simulink model "Neurofeedback_Fuzzy_MISO_Full_3x3"  (R2022a)
settings: Solver=VariableStepAuto  StartTime=0.0  StopTime=2700  RelTol=1e-3
libraries: dspsrcs4 x12, simulink x5, fuzblock x1
(part 1 of 2)
settings Model: Creator=mdls3  LastModifiedBy=mariodelossantos
settings DebuggingCC: SignalRangeChecking=warning  UnderSpecifiedDimensionMsg=warning

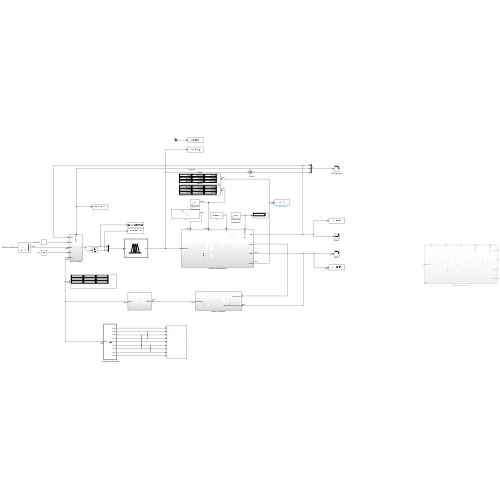
[thumbnail: Simulink's stored preview of the top-level diagram]
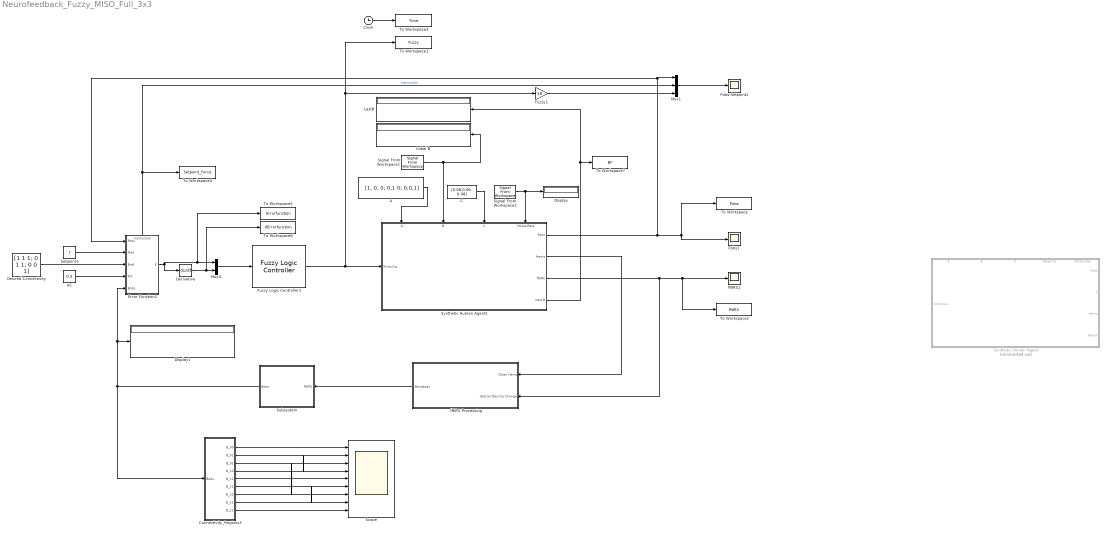
== system Neurofeedback_Fuzzy_MISO_Full_3x3 ==
  A : Constant  Value=[1, 0, 0; 0,1 0; 0,0,1]
  C : Constant  Value=[0.08;0.06; 0.08]
  Clock : Clock
  Connectivity_Regions3 : MATLAB Function  TreatAsAtomicUnit=on
  Derivative : Derivative  CoefficientInTFapproximation=1
  Desired Connectivity : Constant  Value="[1   1  1; 0 1 1; 0 0 1]"
  Display : Display
  Display1 : Display
  Error Function2 : Subsystem
      settings: PortSchema="{\"entries\":[{\"content\":{\"sides\":[{\"content\":{\"connectorIds\":[\"In1\",\"In2\",\"In3\",\"In4\",\"In5\"]},\"type\":\"ConnectorPlacement.EquallySpacedRectSide\",\"uuid\":\"444fbf9f-83f0-405e-b780-73f2a519e5d8\"},{\"content\":{\"connectorIds\":[\"Out1\"],\"side\":\"RIGHT\"},\"type\":\"ConnectorPlacement.EquallySpacedRectSide\",\"uuid\":\"580feeb9-eb76-4e38-ada2-7c0fba9b3602\"},{\"content\":{\"connectorIds\":[\"Out2\"],\"side\":\"TOP\"},\"type\":\"ConnectorPlacement.EquallySpacedRectSide\",\"uuid\":\"86f5bef5-f023-4b75-b93f-dc016b73225e\"}]},\"type\":\"ConnectorPlacement.EquallySpacedConnector\",\"uuid\":\"50bb9fda-b7f3-427b-ab4c-df885dc392aa\"}],\"packageUris\":[\"http://schema.mathworks.com/mf0/Connector/R2020b\"],\"version\":\"1.0\"}"
  Fuzzy Logic Controller1 : fuzblock/Fuzzy Logic  Controller  FIS=cFNIRS_MISO_v4  OutputSampleNumber=101  DataType=double  FuzzifiedInputs=off  RuleFiringStrengths=off  RuleOutputs=off  AggregatedOutputs=off  SimulateUsing=Interpreted execution  OutOfRangeInputValueMessage=warning  NoRuleFiredMessage=warning  EmptyOutputFuzzySetMessage=warning
  Fuzzy1 : Gain  Gain=10
  Initial B : Display
  LastB : Display
  Mux1 : Mux  Inputs=3
  Mux4 : Mux  Inputs=2
  Pobs-Setpoint1 : Scope
  Pobs1 : Scope
  Scope : Scope  NumInputPorts=9
  Setpoint1 : Constant  Value=7
  Signal From Workspace1 : dspsrcs4/Signal From Workspace  X=B  Ts=1  nsamps=1  OutputAfterFinalValue=Setting to zero  ignoreOrWarnInputAndFrameLengths=off  OutputFrames=off
  Signal From Workspace2 : dspsrcs4/Signal From Workspace  X=Noise  Ts=1  nsamps=1  OutputAfterFinalValue=Setting to zero  ignoreOrWarnInputAndFrameLengths=off  OutputFrames=off
  Subsystem : Subsystem
  Synthetic Human Agent : Subsystem  Commented=on
      settings: PortSchema="{\"entries\":[{\"content\":{\"sides\":[{\"content\":{\"connectorIds\":[\"In1\"]},\"type\":\"ConnectorPlacement.EquallySpacedRectSide\",\"uuid\":\"bfbcc5e8-6241-430f-b542-d1842988c81e\"},{\"content\":{\"connectorIds\":[\"Out1\",\"Out2\",\"Out3\",\"Out4\"],\"side\":\"RIGHT\"},\"type\":\"ConnectorPlacement.EquallySpacedRectSide\",\"uuid\":\"5787ae13-1686-4c0f-bd71-92bd424cb6c3\"},{\"content\":{\"connectorIds\":[\"In2\",\"In3\",\"In4\",\"In5\",\"In6\"],\"side\":\"TOP\"},\"type\":\"ConnectorPlacement.EquallySpacedRectSide\",\"uuid\":\"d1dd531e-b262-408a-a912-471f5b03e825\"}]},\"type\":\"ConnectorPlacement.EquallySpacedConnector\",\"uuid\":\"b2c21004-90c2-4258-a219-9564d29dafe7\"}],\"packageUris\":[\"http://schema.mathworks.com/mf0/Connector/R2020b\"],\"version\":\"1.0\"}"
  Synthetic Human Agent1 : Subsystem
      settings: PortSchema="{\"entries\":[{\"content\":{\"sides\":[{\"content\":{\"connectorIds\":[\"In1\"]},\"type\":\"ConnectorPlacement.EquallySpacedRectSide\",\"uuid\":\"bfbcc5e8-6241-430f-b542-d1842988c81e\"},{\"content\":{\"connectorIds\":[\"Out1\",\"Out2\",\"Out3\",\"Out4\"],\"side\":\"RIGHT\"},\"type\":\"ConnectorPlacement.EquallySpacedRectSide\",\"uuid\":\"5787ae13-1686-4c0f-bd71-92bd424cb6c3\"},{\"content\":{\"connectorIds\":[\"In2\",\"In3\",\"In4\",\"In5\"],\"side\":\"TOP\"},\"type\":\"ConnectorPlacement.EquallySpacedRectSide\",\"uuid\":\"d1dd531e-b262-408a-a912-471f5b03e825\"}]},\"type\":\"ConnectorPlacement.EquallySpacedConnector\",\"uuid\":\"b2c21004-90c2-4258-a219-9564d29dafe7\"}],\"packageUris\":[\"http://schema.mathworks.com/mf0/Connector/R2020b\"],\"version\":\"1.0\"}"
  To Workspace : ToWorkspace  VariableName=Pobs  SampleTime=-1
  To Workspace1 : ToWorkspace  VariableName=Fuzzy  SampleTime=-1
  To Workspace2 : ToWorkspace  VariableName=fNIRS  SampleTime=-1
  To Workspace3 : ToWorkspace  VariableName=Time  SampleTime=-1
      settings: Save2DSignal=2-D array (concatenate along first dimension)
  To Workspace4 : ToWorkspace  VariableName=Setpoint_Force  SampleTime=-1
  To Workspace5 : ToWorkspace  VariableName=Errorfunction  SampleTime=-1
  To Workspace6 : ToWorkspace  VariableName=dErrorfunction  SampleTime=-1
  To Workspace7 : ToWorkspace  VariableName=BF  SampleTime=-1
  fNIRS Processing : Subsystem
  fNIRS1 : Scope
  w1 : Constant  Value=0.5
  wires:
  Mux1/1 -> Pobs-Setpoint1/1
  Error Function2/1(E) -> Mux4/1, To Workspace5/1, Derivative/1
  Fuzzy1/1 -> Mux1/3
  Synthetic Human Agent1/2(Hemo) -> fNIRS Processing/1(Clean Hemo)
  Derivative/1 -> To Workspace6/1, Mux4/2
  Setpoint1/1 -> Error Function2/2(Pref)
  Error Function2/2(Instruction) -> Mux1/2, To Workspace4/1  "Instruction"
  Synthetic Human Agent1/1(Pobs) -> Error Function2/1(Pobs), Mux1/1, To Workspace/1, Pobs1/1
  Mux4/1 -> Fuzzy Logic Controller1/1
  A/1 -> Synthetic Human Agent1/2(A)
  w1/1 -> Error Function2/4(W1)
  Desired Connectivity/1 -> Error Function2/3(Bref)
  C/1 -> Synthetic Human Agent1/4(C)
  Fuzzy Logic Controller1/1 -> To Workspace1/1, Fuzzy1/1, Synthetic Human Agent1/1(Stimulus)
  Clock/1 -> To Workspace3/1
  Synthetic Human Agent1/4(New B) -> To Workspace7/1, LastB/1
  Signal From Workspace1/1 -> Initial B/1, Synthetic Human Agent1/3(B)
  Signal From Workspace2/1 -> Display/1, Synthetic Human Agent1/5(Noise-Rate)
  Subsystem/1(Bobs) -> Connectivity_Regions3/1(Bobs), Error Function2/5(Bobs), Display1/1
  Synthetic Human Agent1/3(fNIRS) -> fNIRS1/1, To Workspace2/1, fNIRS Processing/2(Optical Density Changes)
  Connectivity_Regions3/1(B_00) -> Scope/1
  Connectivity_Regions3/2(B_01) -> Scope/4
  Connectivity_Regions3/3(B_02) -> Scope/7
  Connectivity_Regions3/4(B_10) -> Scope/2
  Connectivity_Regions3/5(B_11) -> Scope/5
  Connectivity_Regions3/6(B_12) -> Scope/8
  Connectivity_Regions3/7(B_20) -> Scope/3
  Connectivity_Regions3/8(B_21) -> Scope/6
  Connectivity_Regions3/9(B_22) -> Scope/9
  fNIRS Processing/1(Bandpass) -> Subsystem/1(fNIRS)

== system Neurofeedback_Fuzzy_MISO_Full_3x3/Error Function2 ==
  Pobs : Inport
  Pref : Inport  Port=2
  Bref : Inport  Port=3
  W1 : Inport  Port=4
  Bobs : Inport  Port=5
  Error Function : Subsystem
  Rehabilitation Train : Subsystem
  E : Outport
  Instruction : Outport  Port=2
  wires:
  Bref/1 -> Error Function/3(Bref)
  Bobs/1 -> Error Function/4(Bobs)
  W1/1 -> Error Function/5(W1)
  Pref/1 -> Rehabilitation Train/1(In1)
  Pobs/1 -> Error Function/1(Pobs)
  Rehabilitation Train/1(Instruction) -> Instruction/1, Error Function/2(Pref)
  Error Function/1(E) -> E/1

== system Neurofeedback_Fuzzy_MISO_Full_3x3/Subsystem ==
  fNIRS : Inport
  DQ1 : Scope
  Incremental_Avg_Boot1 : Subsystem
  Threshold : Constant  Value=0.5
  getConnectivity_Validation1 : MATLAB Function  TreatAsAtomicUnit=on  SystemSampleTime=0
  Bobs : Outport
  wires:
  getConnectivity_Validation1/2(DQ) -> DQ1/1
  Incremental_Avg_Boot1/1("D ") -> getConnectivity_Validation1/1("D ")
  Threshold/1 -> getConnectivity_Validation1/2(Threshold)
  fNIRS/1 -> Incremental_Avg_Boot1/1(fNIRS)
  getConnectivity_Validation1/1(Bobs) -> Bobs/1

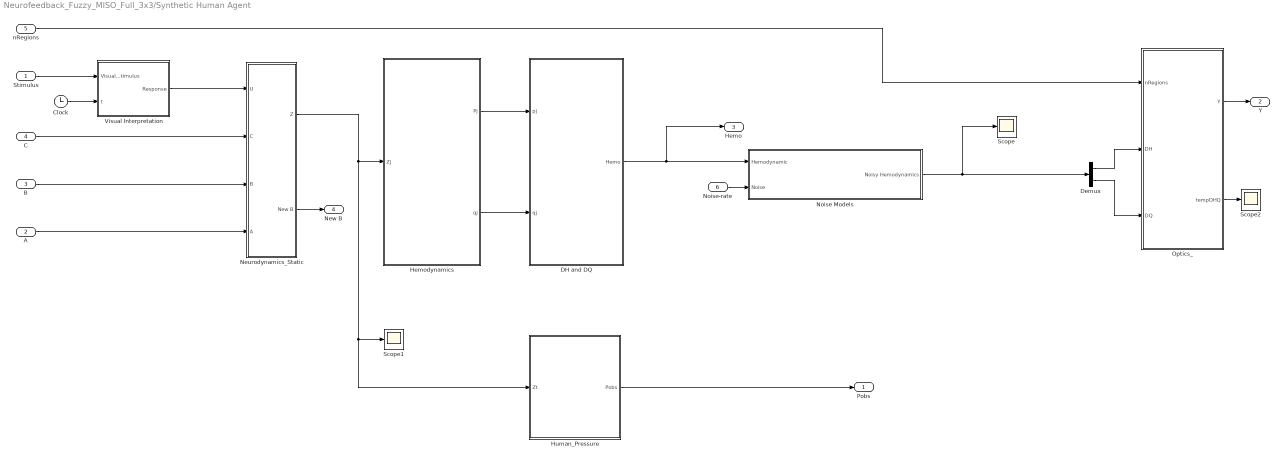
== system Neurofeedback_Fuzzy_MISO_Full_3x3/Synthetic Human Agent ==
  Stimulus : Inport
  A : Inport  Port=2
  B : Inport  Port=3
  C : Inport  Port=4
  nRegions : Inport  Port=5
  Noise-rate : Inport  Port=6
  Clock : Clock
  DH and DQ : Subsystem
  Demux : Demux  Outputs=2
  Hemodynamics : Subsystem
  Human_Pressure : Subsystem
  Neurodynamics_Static : Subsystem
  Noise Models : Subsystem
  Optics_ : MATLAB Function  TreatAsAtomicUnit=on
  Scope : Scope
  Scope1 : Scope
  Scope2 : Scope
  Visual Interpretation : MATLAB Function  TreatAsAtomicUnit=on
  Pobs : Outport
  Y : Outport  Port=2
  Hemo : Outport  Port=3
  New B : Outport  Port=4
  wires:
  DH and DQ/1(Hemo) -> Hemo/1, Noise Models/1(Hemodynamic)
  Hemodynamics/1(Pj) -> DH and DQ/1(pj)
  C/1 -> Neurodynamics_Static/2(C)
  Hemodynamics/2(qj) -> DH and DQ/2(qj)
  A/1 -> Neurodynamics_Static/4(A)
  Human_Pressure/1(Pobs) -> Pobs/1
  B/1 -> Neurodynamics_Static/3(B)
  Neurodynamics_Static/1(Z) -> Scope1/1, Human_Pressure/1(Zt), Hemodynamics/1(Zj)
  Clock/1 -> Visual Interpretation/2(t)
  Stimulus/1 -> Visual Interpretation/1(Visual_Stimulus)
  Visual Interpretation/1(Response) -> Neurodynamics_Static/1(U)
  Noise Models/1(Noisy Hemodynamics) -> Scope/1, Demux/1
  Noise-rate/1 -> Noise Models/2(Noise)
  Demux/1 -> Optics_/2(DH)
  Demux/2 -> Optics_/3(DQ)
  Optics_/1(Y) -> Y/1
  nRegions/1 -> Optics_/1(nRegions)
  Optics_/2(tempDHQ) -> Scope2/1
  Neurodynamics_Static/2(New B) -> New B/1

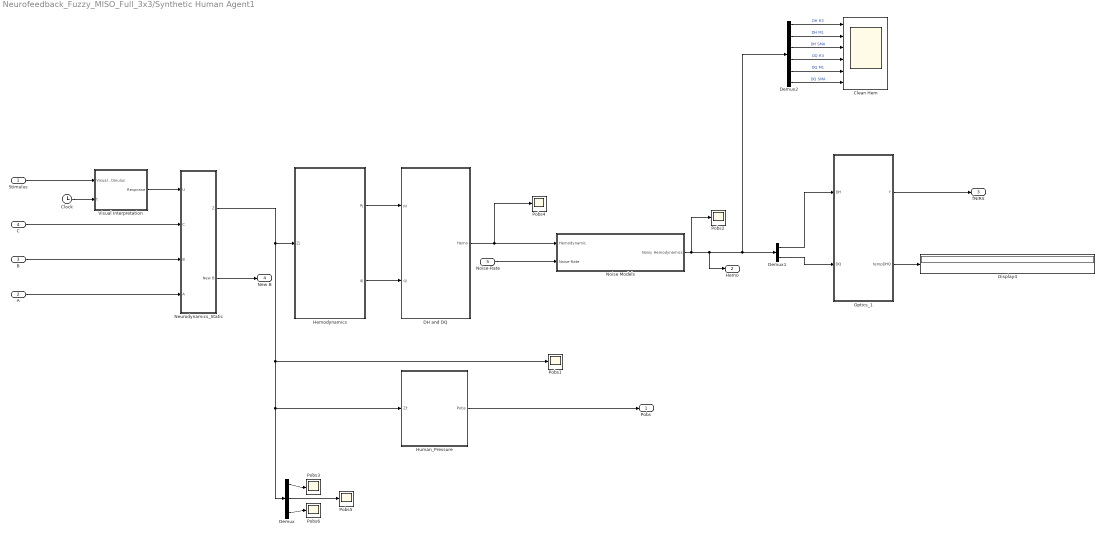
== system Neurofeedback_Fuzzy_MISO_Full_3x3/Synthetic Human Agent1 ==
  Stimulus : Inport
  A : Inport  Port=2
  B : Inport  Port=3
  C : Inport  Port=4
  Noise-Rate : Inport  Port=5
  Clean Hem : Scope  NumInputPorts=6
  Clock : Clock
  DH and DQ : Subsystem
  Demux : Demux  Outputs=3
  Demux1 : Demux  Outputs=2
  Demux2 : Demux  Outputs=6
  Display4 : Display
  Hemodynamics : Subsystem
  Human_Pressure : Subsystem
  Neurodynamics_Static : Subsystem
  Noise Models : Subsystem
  Optics_1 : MATLAB Function  TreatAsAtomicUnit=on
  Pobs{1..6} (6 alike) : Scope
  Visual Interpretation : MATLAB Function  TreatAsAtomicUnit=on
  Pobs : Outport
  Hemo : Outport  Port=2
  fNIRS : Outport  Port=3
  New B : Outport  Port=4
  wires:
  DH and DQ/1(Hemo) -> Pobs4/1, Noise Models/1(Hemodynamic)
  C/1 -> Neurodynamics_Static/2(C)
  A/1 -> Neurodynamics_Static/4(A)
  Human_Pressure/1(Pobs) -> Pobs/1
  B/1 -> Neurodynamics_Static/3(B)
  Demux1/1 -> Optics_1/1(DH)
  Demux1/2 -> Optics_1/2(DQ)
  Optics_1/1(Y) -> fNIRS/1
  Noise-Rate/1 -> Noise Models/2(Noise-Rate)
  Noise Models/1(Noisy Hemodynamics) -> Pobs2/1, Hemo/1, Demux2/1, Demux1/1
  Optics_1/2(tempDHQ) -> Display4/1
  Hemodynamics/1(Pj) -> DH and DQ/1(pj)
  Hemodynamics/2(qj) -> DH and DQ/2(qj)
  Demux2/2 -> Clean Hem/2  "DH M1"
  Demux2/1 -> Clean Hem/1  "DH R3"
  Demux2/3 -> Clean Hem/3  "DH SMA"
  Demux2/4 -> Clean Hem/4  "DQ R3"
  Demux2/5 -> Clean Hem/5  "DQ M1"
  Demux2/6 -> Clean Hem/6  "DQ SMA"
  Clock/1 -> Visual Interpretation/2(t)
  Stimulus/1 -> Visual Interpretation/1(Visual_Stimulus)
  Visual Interpretation/1(Response) -> Neurodynamics_Static/1(U)
  Neurodynamics_Static/2(New B) -> New B/1
  Demux/1 -> Pobs3/1
  Demux/2 -> Pobs5/1
  Demux/3 -> Pobs6/1
  Neurodynamics_Static/1(Z) -> Pobs1/1, Demux/1, Human_Pressure/1(Zt), Hemodynamics/1(Zj)

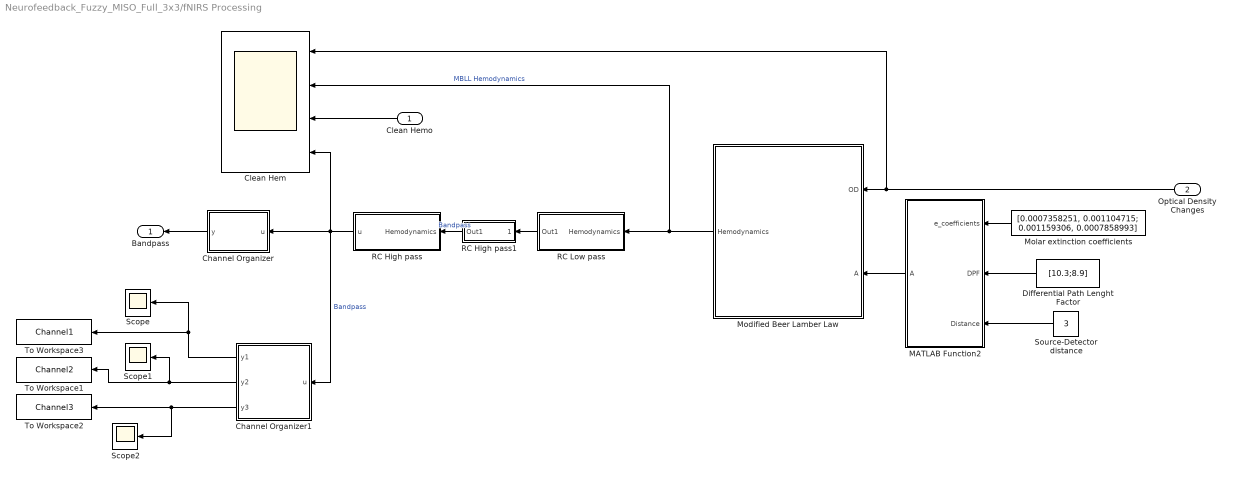
== system Neurofeedback_Fuzzy_MISO_Full_3x3/fNIRS Processing ==
  Clean Hemo : Inport
  Optical Density Changes : Inport  Port=2
  Channel Organizer : MATLAB Function  TreatAsAtomicUnit=on
  Channel Organizer1 : MATLAB Function  TreatAsAtomicUnit=on
  Clean Hem : Scope  NumInputPorts=4
  Differential Path Lenght Factor : Constant  Value=[10.3;8.9]
  MATLAB Function2 : MATLAB Function  TreatAsAtomicUnit=on
  Modified Beer Lamber Law : MATLAB Function  TreatAsAtomicUnit=on
  Molar extinction coefficients : Constant  Value=|
      | [0.0007358251, 0.001104715;
      | 0.001159306, 0.0007858993]
  RC High pass : Subsystem
  RC High pass1 : Subsystem
  RC Low pass : Subsystem
  Scope : Scope
  Scope1 : Scope
  Scope2 : Scope
  Source-Detector distance : Constant  Value=3
  To Workspace1 : ToWorkspace  VariableName=Channel2  SaveFormat=Structure With Time  SampleTime=-1
  To Workspace2 : ToWorkspace  VariableName=Channel3  SaveFormat=Structure With Time  SampleTime=-1
  To Workspace3 : ToWorkspace  VariableName=Channel1  SaveFormat=Structure With Time  SampleTime=-1
  Bandpass : Outport
  wires:
  Modified Beer Lamber Law/1(Hemodynamics) -> RC Low pass/1(Hemodynamics), Clean Hem/2  "MBLL Hemodynamics"
  Optical Density Changes/1 -> Clean Hem/1, Modified Beer Lamber Law/1(OD)
  RC High pass/1(u) -> Channel Organizer/1(u), Channel Organizer1/1(u), Clean Hem/4  "Bandpass"
  MATLAB Function2/1(A) -> Modified Beer Lamber Law/2(A)
  RC Low pass/1(Out1) -> RC High pass1/1(Hemodynamics)
  Clean Hemo/1 -> Clean Hem/3
  RC High pass1/1(Out1) -> RC High pass/1(Hemodynamics)  "Bandpass"
  Channel Organizer1/1(y1) -> Scope/1, To Workspace3/1
  Channel Organizer1/2(y2) -> Scope1/1, To Workspace1/1
  Channel Organizer1/3(y3) -> Scope2/1, To Workspace2/1
  Source-Detector distance/1 -> MATLAB Function2/3(Distance)
  Differential Path Lenght Factor/1 -> MATLAB Function2/2(DPF)
  Molar extinction coefficients/1 -> MATLAB Function2/1(e_coefficients)
  Channel Organizer/1(y) -> Bandpass/1

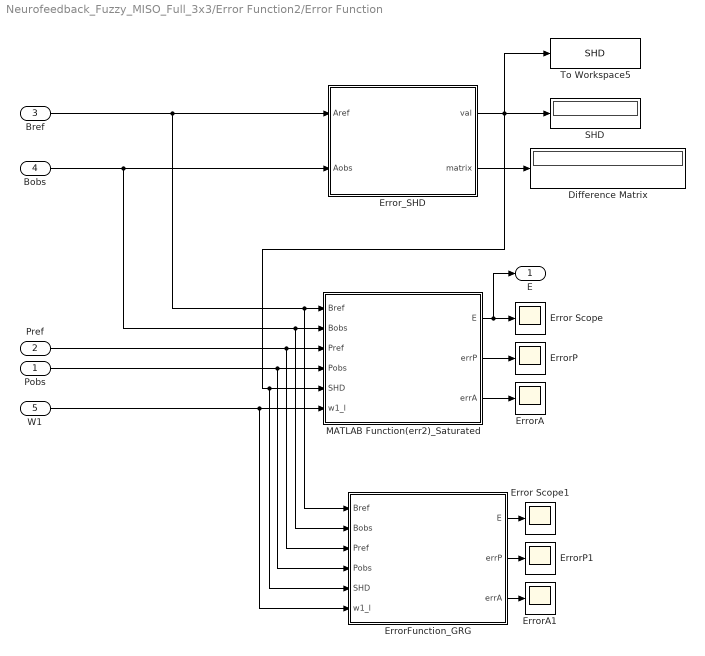
== system Neurofeedback_Fuzzy_MISO_Full_3x3/Error Function2/Error Function ==
  Pobs : Inport
  Pref : Inport  Port=2
  Bref : Inport  Port=3
  Bobs : Inport  Port=4
  W1 : Inport  Port=5
  Difference Matrix : Display
  Error Scope : Scope
  Error Scope1 : Scope
  ErrorA : Scope
  ErrorA1 : Scope
  ErrorFunction_GRG : MATLAB Function  TreatAsAtomicUnit=on
  ErrorP : Scope
  ErrorP1 : Scope
  Error_SHD : MATLAB Function  TreatAsAtomicUnit=on
  MATLAB Function(err2)_Saturated : MATLAB Function  TreatAsAtomicUnit=on
  SHD : Display
  To Workspace5 : ToWorkspace  VariableName=SHD  SampleTime=-1
  E : Outport
  wires:
  Error_SHD/2(matrix) -> Difference Matrix/1
  Bref/1 -> ErrorFunction_GRG/1(Bref), MATLAB Function(err2)_Saturated/1(Bref), Error_SHD/1(Aref)
  Error_SHD/1(val) -> To Workspace5/1, ErrorFunction_GRG/5(SHD), MATLAB Function(err2)_Saturated/5(SHD), SHD/1
  Bobs/1 -> ErrorFunction_GRG/2(Bobs), MATLAB Function(err2)_Saturated/2(Bobs), Error_SHD/2(Aobs)
  Pref/1 -> ErrorFunction_GRG/3(Pref), MATLAB Function(err2)_Saturated/3(Pref)
  W1/1 -> MATLAB Function(err2)_Saturated/6(w1_l), ErrorFunction_GRG/6(w1_l)
  MATLAB Function(err2)_Saturated/1(E) -> E/1, Error Scope/1
  Pobs/1 -> ErrorFunction_GRG/4(Pobs), MATLAB Function(err2)_Saturated/4(Pobs)
  MATLAB Function(err2)_Saturated/2(errP) -> ErrorP/1
  MATLAB Function(err2)_Saturated/3(errA) -> ErrorA/1
  ErrorFunction_GRG/2(errP) -> ErrorP1/1
  ErrorFunction_GRG/3(errA) -> ErrorA1/1
  ErrorFunction_GRG/1(E) -> Error Scope1/1

== system Neurofeedback_Fuzzy_MISO_Full_3x3/Error Function2/Rehabilitation Train ==
  In1 : Inport
  Duty_Cycle_U1 : Constant  Value=0.1666666666666667  OutMin=[0]  OutMax=[0.8]
  Period_Time_U1 : Constant  Value=30
  Setpoint_follow : Product
  Variable Pulse Generator2 : VariablePulseGenerator  AllowZeroPulseWidth=on  RunAtFixedTimeIntervals=on  SampleTime=1/10
  Instruction : Outport
  wires:
  Duty_Cycle_U1/1 -> Variable Pulse Generator2/1
  In1/1 -> Setpoint_follow/2
  Period_Time_U1/1 -> Variable Pulse Generator2/2
  Setpoint_follow/1 -> Instruction/1
  Variable Pulse Generator2/1 -> Setpoint_follow/1

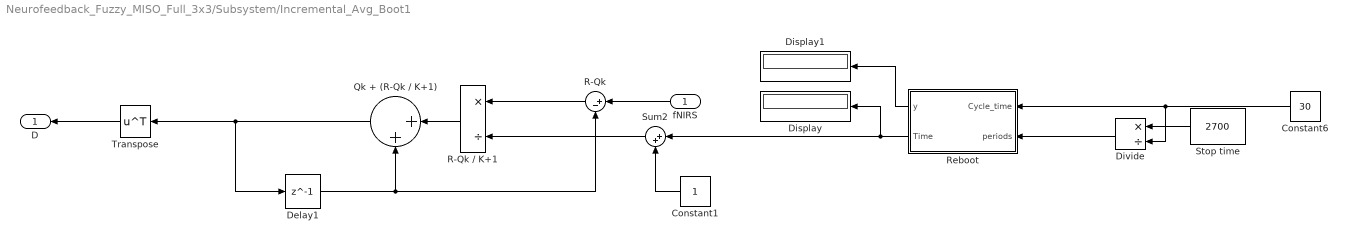
== system Neurofeedback_Fuzzy_MISO_Full_3x3/Subsystem/Incremental_Avg_Boot1 ==
  fNIRS : Inport
  Constant1 : Constant
  Constant6 : Constant  Value=30
  Delay1 : Delay  DelayLength=1  InitialCondition=[0; 0; 0; 0;0;0]
  Display : Display
  Display1 : Display
  Divide : Product  Inputs=*/
  "Qk + (R-Qk / K+1) " : Sum  Inputs=|++
  R-Qk : Sum  Inputs=|+-
  R-Qk / K+1 : Product  Inputs=*/
  Reboot : Subsystem
  Stop time : Constant  Value=2700
  Sum2 : Sum  Inputs=|++
  Transpose : Math  Operator=transpose
  "D " : Outport
  wires:
  Constant1/1 -> Sum2/2
  fNIRS/1 -> R-Qk/1
  R-Qk / K+1/1 -> "Qk + (R-Qk / K+1) "/1
  Sum2/1 -> R-Qk / K+1/2
  R-Qk/1 -> R-Qk / K+1/1
  Delay1/1 -> R-Qk/2, "Qk + (R-Qk / K+1) "/2
  Reboot/2(Time) -> Sum2/1, Display/1
  Constant6/1 -> Reboot/1(Cycle_time), Divide/2
  Reboot/1(y) -> Display1/1
  Divide/1 -> Reboot/2(periods)
  Stop time/1 -> Divide/1
  "Qk + (R-Qk / K+1) "/1 -> Transpose/1, Delay1/1
  Transpose/1 -> "D "/1

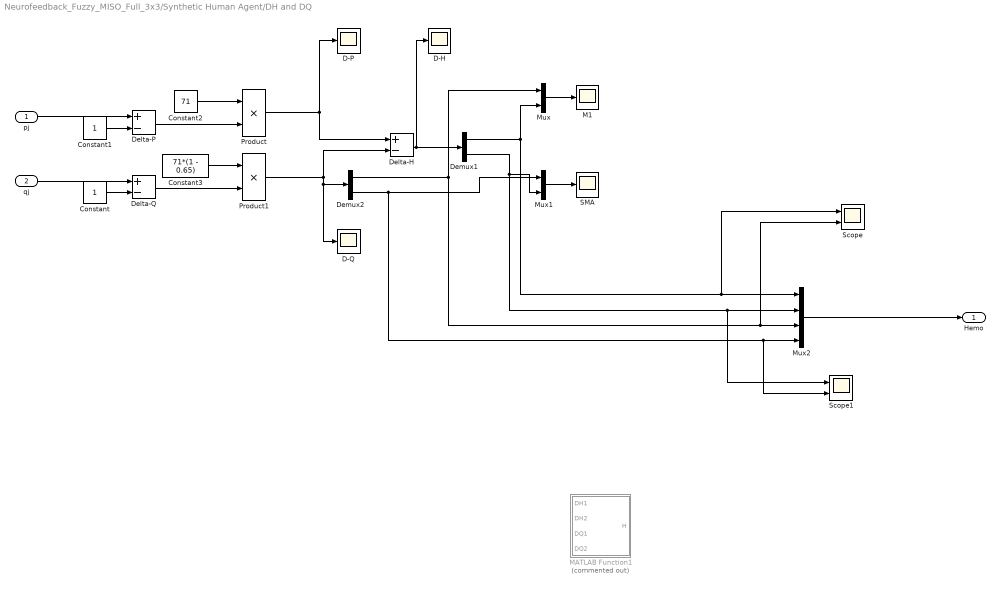
== system Neurofeedback_Fuzzy_MISO_Full_3x3/Synthetic Human Agent/DH and DQ ==
  pj : Inport
  qj : Inport  Port=2
  Constant : Constant
  Constant1 : Constant
  Constant2 : Constant  Value=71
  Constant3 : Constant  Value=71*(1 - 0.65)
  D-H : Scope
  D-P : Scope
  D-Q : Scope
  Delta-H : Sum  Inputs=+-
  Delta-P : Sum  Inputs=+-
  Delta-Q : Sum  Inputs=+-
  Demux1 : Demux  Outputs=2
  Demux2 : Demux  Outputs=2
  M1 : Scope
  MATLAB Function1 : MATLAB Function  Commented=on  TreatAsAtomicUnit=on
  Mux : Mux  Inputs=2
  Mux1 : Mux  Inputs=2
  Mux2 : Mux
  Product : Product
  Product1 : Product
  SMA : Scope
  Scope : Scope  NumInputPorts=2
  Scope1 : Scope  NumInputPorts=2
  Hemo : Outport
  wires:
  Constant2/1 -> Product/1
  Delta-Q/1 -> Product1/2
  Constant3/1 -> Product1/1
  Demux2/2 -> Mux1/1, Scope1/2, Mux2/4
  pj/1 -> Delta-P/1
  Mux1/1 -> SMA/1
  Mux/1 -> M1/1
  Constant/1 -> Delta-Q/2
  Delta-P/1 -> Product/2
  Product1/1 -> Demux2/1, D-Q/1, Delta-H/2
  qj/1 -> Delta-Q/1
  Delta-H/1 -> Demux1/1, D-H/1
  Demux1/1 -> Scope/1, Mux2/1, Mux/2
  Demux1/2 -> Scope1/1, Mux2/2, Mux1/2
  Product/1 -> D-P/1, Delta-H/1
  Demux2/1 -> Mux/1, Scope/2, Mux2/3
  Constant1/1 -> Delta-P/2
  Mux2/1 -> Hemo/1

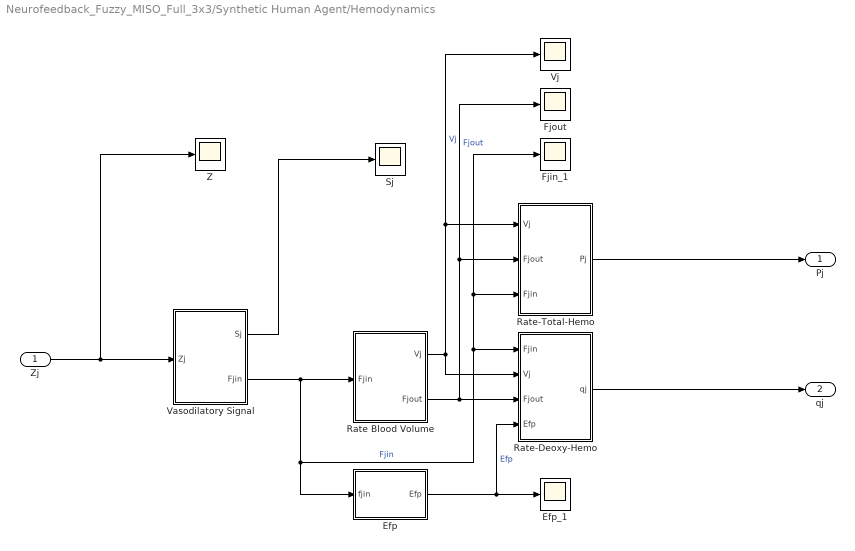
== system Neurofeedback_Fuzzy_MISO_Full_3x3/Synthetic Human Agent/Hemodynamics ==
  Zj : Inport
  Efp : MATLAB Function  TreatAsAtomicUnit=on
  Efp_1 : Scope
  Fjin_1 : Scope
  Fjout : Scope
  Rate Blood Volume : Subsystem
  Rate-Deoxy-Hemo : Subsystem
  Rate-Total-Hemo : Subsystem
  Sj : Scope
  Vasodilatory Signal : Subsystem
  Vj : Scope
  Z : Scope
  Pj : Outport
  qj : Outport  Port=2
  wires:
  Rate-Deoxy-Hemo/1(qj) -> qj/1
  Zj/1 -> Vasodilatory Signal/1(Zj), Z/1
  Vasodilatory Signal/1(Sj) -> Sj/1
  Rate Blood Volume/2(Fjout) -> Fjout/1, Rate-Total-Hemo/2(Fjout), Rate-Deoxy-Hemo/3(Fjout)  "Fjout"
  Rate Blood Volume/1(Vj) -> Vj/1, Rate-Total-Hemo/1(Vj), Rate-Deoxy-Hemo/2(Vj)  "Vj"
  Rate-Total-Hemo/1(Pj) -> Pj/1
  Efp/1(Efp) -> Rate-Deoxy-Hemo/4(Efp), Efp_1/1  "Efp"
  Vasodilatory Signal/2(Fjin) -> Efp/1(fjin), Fjin_1/1, Rate-Total-Hemo/3(Fjin), Rate-Deoxy-Hemo/1(Fjin), Rate Blood Volume/1(Fjin)  "Fjin"

== system Neurofeedback_Fuzzy_MISO_Full_3x3/Synthetic Human Agent/Human_Pressure ==
  Zt : Inport
  Clock : Clock
  Gain : Gain  Gain=10
  Pressure Generator : MATLAB Function  TreatAsAtomicUnit=on
  SENSOR : MATLAB Function  TreatAsAtomicUnit=on
  Scope : Scope
  Scope1 : Scope
  Pobs : Outport
  wires:
  Clock/1 -> Pressure Generator/2(t)
  Zt/1 -> Pressure Generator/1(Zt)
  SENSOR/1(Pobs) -> Scope1/1, Gain/1
  Pressure Generator/1(Pobs) -> SENSOR/1(Vout), Scope/1
  Gain/1 -> Pobs/1

== system Neurofeedback_Fuzzy_MISO_Full_3x3/Synthetic Human Agent/Neurodynamics_Static ==
  U : Inport
  C : Inport  Port=2
  B : Inport  Port=3
  A : Inport  Port=4
  B_Dynamic : Subsystem
  Clock : Clock
  Integrator : Integrator
  Jt : MATLAB Function  TreatAsAtomicUnit=on
  Product1 : Product  Multiplication=Matrix(*)
  Sum : Sum  Inputs=|++
  Z : Outport
  New B : Outport  Port=2
  wires:
  Integrator/1 -> Jt/1(Zt), Z/1
  Product1/1 -> Sum/1
  Jt/1(Jt) -> Sum/2
  Sum/1 -> Integrator/1
  U/1 -> Product1/2, B_Dynamic/1(U), Jt/2(U)
  C/1 -> Product1/1
  A/1 -> Jt/4(A_input)
  Clock/1 -> B_Dynamic/3(T)
  B/1 -> B_Dynamic/2(B)
  B_Dynamic/1(B_d) -> New B/1, Jt/3(B_input)

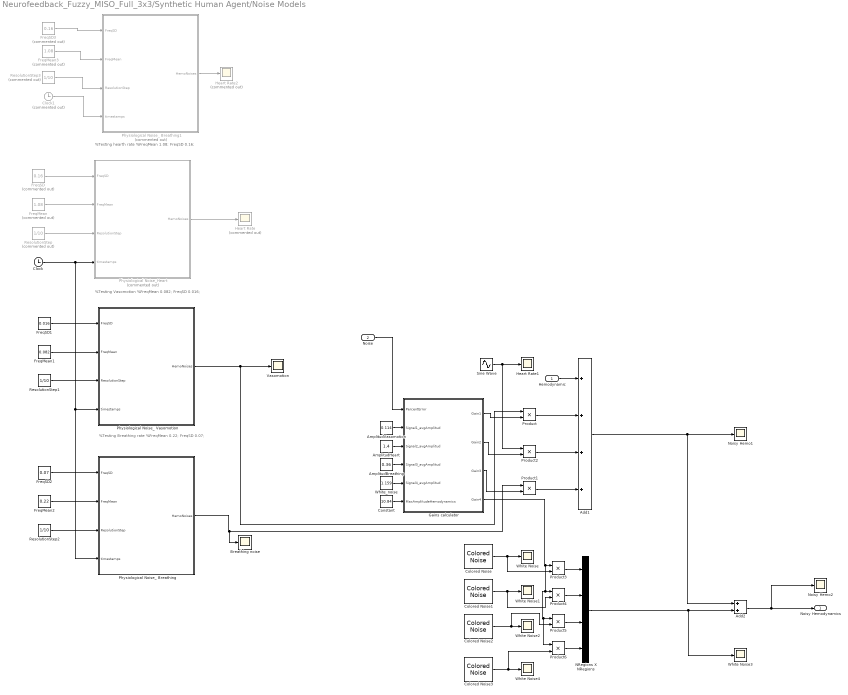
== system Neurofeedback_Fuzzy_MISO_Full_3x3/Synthetic Human Agent/Noise Models ==
  note: %Testing hearth rate
      | %FreqMean 1.08; FreqSD 0.16;
  note: %Testing Breathing rate
      | %FreqMean 0.22; FreqSD 0.07;
  note: %Testing Vasomotion
      | %FreqMean 0.082; FreqSD 0.016;
  Hemodynamic : Inport
  Noise : Inport  Port=2
  Add1 : Sum  Inputs=++++
  Add2 : Sum
  AmplitudBreathing : Constant  Value=0.36
  AmplitudHeart : Constant  Value=1.4
  AmplitudVasomotion : Constant  Value=0.114
  Breathing noise : Scope
  Clock : Clock
  Clock1 : Clock  Commented=on
  Colored Noise : dspsrcs4/Colored Noise  Color=white  InverseFrequencyPower=1  BoundedOutput=on  NumChannels=1  OutputDataType=double  SamplesPerFrame=1  SampleTime=1/10  RandomStream=mt19937ar with seed  Seed=67  SimulateUsing=Interpreted execution
      settings: SourceProductBaseCode=DS
  Colored Noise1 : dspsrcs4/Colored Noise  Color=white  InverseFrequencyPower=1  BoundedOutput=on  NumChannels=1  OutputDataType=double  SamplesPerFrame=1  SampleTime=1/10  RandomStream=mt19937ar with seed  Seed=40  SimulateUsing=Interpreted execution
      settings: SourceProductBaseCode=DS
  Colored Noise2 : dspsrcs4/Colored Noise  Color=white  InverseFrequencyPower=1  BoundedOutput=on  NumChannels=1  OutputDataType=double  SamplesPerFrame=1  SampleTime=1/10  RandomStream=mt19937ar with seed  Seed=41  SimulateUsing=Interpreted execution
      settings: SourceProductBaseCode=DS
  Colored Noise3 : dspsrcs4/Colored Noise  Color=white  InverseFrequencyPower=1  BoundedOutput=on  NumChannels=1  OutputDataType=double  SamplesPerFrame=1  SampleTime=1/10  RandomStream=mt19937ar with seed  Seed=50  SimulateUsing=Interpreted execution
      settings: SourceProductBaseCode=DS
  Constant : Constant  Value=10.84
  FreqMean : Constant  Commented=on  Value=1.08
  FreqMean1 : Constant  Value=0.082
  FreqMean2 : Constant  Value=0.22
  FreqMean3 : Constant  Commented=on  Value=1.08
  FreqSD : Constant  Commented=on  Value=0.16
  FreqSD1 : Constant  Value=0.016
  FreqSD2 : Constant  Value=0.07
  FreqSD3 : Constant  Commented=on  Value=0.16
  Gains calculator : MATLAB Function  TreatAsAtomicUnit=on
  Heart Rate : Scope  Commented=on
  Heart Rate1 : Scope
  Heart Rate2 : Scope  Commented=on
  NRegions X NRegions : Mux
  Noisy Hemo1 : Scope
  Noisy Hemo2 : Scope
  Physiological Noise_ Breathing : MATLAB Function  TreatAsAtomicUnit=on
  Physiological Noise_ Breathing1 : MATLAB Function  Commented=on  TreatAsAtomicUnit=on
  Physiological Noise_ Vasomotion : MATLAB Function  TreatAsAtomicUnit=on
  Physiological Noise_Heart : MATLAB Function  Commented=on  TreatAsAtomicUnit=on
  Product{,1..6} (7 alike) : Product
  ResolutionStep : Constant  Commented=on  Value=1/10
  ResolutionStep1 : Constant  Value=1/10
  ResolutionStep2 : Constant  Value=1/10
  ResolutionStep3 : Constant  Commented=on  Value=1/10
  Sine Wave : Sin  Frequency=1.08 * 2*pi  SampleTime=0
  Vasomotion : Scope
  White Noise{,1..4} (5 alike) : Scope
  White_noise : Constant  Value=1.159
  Noisy Hemodynamics : Outport
  wires:
  FreqSD/1 -> Physiological Noise_Heart/1(FreqSD)
  FreqMean/1 -> Physiological Noise_Heart/2(FreqMean)
  ResolutionStep/1 -> Physiological Noise_Heart/3(ResolutionStep)
  ResolutionStep1/1 -> Physiological Noise_ Vasomotion/3(ResolutionStep)
  FreqSD1/1 -> Physiological Noise_ Vasomotion/1(FreqSD)
  Clock/1 -> Physiological Noise_Heart/4(timestamps), Physiological Noise_ Breathing/4(timestamps), Physiological Noise_ Vasomotion/4(timestamps)
  FreqMean1/1 -> Physiological Noise_ Vasomotion/2(FreqMean)
  Physiological Noise_ Breathing/1(HemoNoises) -> Product1/1, Breathing noise/1
  ResolutionStep2/1 -> Physiological Noise_ Breathing/3(ResolutionStep)
  FreqMean2/1 -> Physiological Noise_ Breathing/2(FreqMean)
  FreqSD2/1 -> Physiological Noise_ Breathing/1(FreqSD)
  Physiological Noise_ Vasomotion/1(HemoNoises) -> Product/1, Vasomotion/1
  Physiological Noise_Heart/1(HemoNoises) -> Heart Rate/1
  Physiological Noise_ Breathing1/1(HemoNoises) -> Heart Rate2/1
  Clock1/1 -> Physiological Noise_ Breathing1/4(timestamps)
  FreqSD3/1 -> Physiological Noise_ Breathing1/1(FreqSD)
  FreqMean3/1 -> Physiological Noise_ Breathing1/2(FreqMean)
  ResolutionStep3/1 -> Physiological Noise_ Breathing1/3(ResolutionStep)
  Sine Wave/1 -> Product2/1, Heart Rate1/1
  Gains calculator/1(Gain1) -> Product/2
  Add1/1 -> Add2/1, Noisy Hemo1/1
  AmplitudVasomotion/1 -> Gains calculator/2(Signal1_avgAmplitud)
  Hemodynamic/1 -> Add1/1
  Constant/1 -> Gains calculator/6(MaxAmplitudeHemodynamics)
  Gains calculator/2(Gain2) -> Product2/2
  Gains calculator/3(Gain3) -> Product1/2
  AmplitudHeart/1 -> Gains calculator/3(Signal2_avgAmplitud)
  AmplitudBreathing/1 -> Gains calculator/4(Signal3_avgAmplitud)
  Colored Noise/1 -> Product3/2, White Noise/1
  Colored Noise1/1 -> Product4/2, White Noise1/1
  Colored Noise2/1 -> Product5/2, White Noise2/1
  NRegions X NRegions/1 -> White Noise3/1, Add2/2
  Colored Noise3/1 -> Product6/2, White Noise4/1
  Add2/1 -> Noisy Hemodynamics/1, Noisy Hemo2/1
  Product/1 -> Add1/2
  Product2/1 -> Add1/3
  Product1/1 -> Add1/4
  Product3/1 -> NRegions X NRegions/1
  White_noise/1 -> Gains calculator/5(Signal4_avgAmplitud)
  Gains calculator/4(Gain4) -> Product6/1, Product5/1, Product4/1, Product3/1
  Product4/1 -> NRegions X NRegions/2
  Product5/1 -> NRegions X NRegions/3
  Product6/1 -> NRegions X NRegions/4
  Noise/1 -> Gains calculator/1(PercentError)

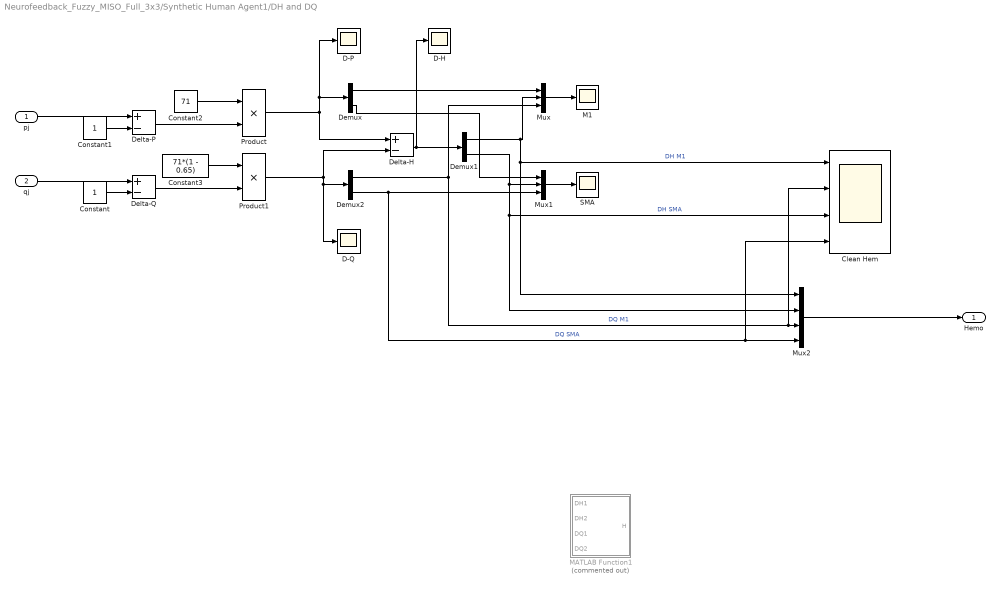
== system Neurofeedback_Fuzzy_MISO_Full_3x3/Synthetic Human Agent1/DH and DQ ==
  pj : Inport
  qj : Inport  Port=2
  Clean Hem : Scope  NumInputPorts=4
  Constant : Constant
  Constant1 : Constant
  Constant2 : Constant  Value=71
  Constant3 : Constant  Value=71*(1 - 0.65)
  D-H : Scope
  D-P : Scope
  D-Q : Scope
  Delta-H : Sum  Inputs=+-
  Delta-P : Sum  Inputs=+-
  Delta-Q : Sum  Inputs=+-
  Demux : Demux  Outputs=2
  Demux1 : Demux  Outputs=2
  Demux2 : Demux  Outputs=2
  M1 : Scope
  MATLAB Function1 : MATLAB Function  Commented=on  TreatAsAtomicUnit=on
  Mux : Mux  Inputs=3
  Mux1 : Mux  Inputs=3
  Mux2 : Mux
  Product : Product
  Product1 : Product
  SMA : Scope
  Hemo : Outport
  wires:
  Constant2/1 -> Product/1
  Delta-Q/1 -> Product1/2
  Constant3/1 -> Product1/1
  Demux2/2 -> Clean Hem/4, Mux2/4, Mux1/3  "DQ SMA"
  pj/1 -> Delta-P/1
  Mux1/1 -> SMA/1
  Demux/2 -> Mux1/1
  Mux/1 -> M1/1
  Constant/1 -> Delta-Q/2
  Delta-P/1 -> Product/2
  Product1/1 -> Demux2/1, D-Q/1, Delta-H/2
  qj/1 -> Delta-Q/1
  Demux/1 -> Mux/1
  Delta-H/1 -> Demux1/1, D-H/1
  Demux1/1 -> Mux2/1, Clean Hem/1, Mux/2  "DH M1"
  Demux1/2 -> Clean Hem/3, Mux2/2, Mux1/2  "DH SMA"
  Product/1 -> Demux/1, D-P/1, Delta-H/1
  Demux2/1 -> Clean Hem/2, Mux2/3, Mux/3  "DQ M1"
  Constant1/1 -> Delta-P/2
  Mux2/1 -> Hemo/1

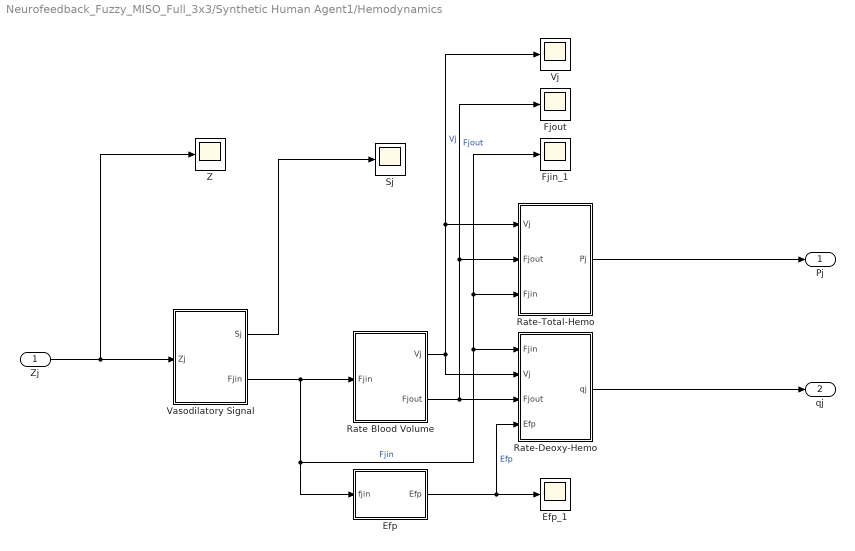
== system Neurofeedback_Fuzzy_MISO_Full_3x3/Synthetic Human Agent1/Hemodynamics ==
  Zj : Inport
  Efp : MATLAB Function  TreatAsAtomicUnit=on
  Efp_1 : Scope
  Fjin_1 : Scope
  Fjout : Scope
  Rate Blood Volume : Subsystem
  Rate-Deoxy-Hemo : Subsystem
  Rate-Total-Hemo : Subsystem
  Sj : Scope
  Vasodilatory Signal : Subsystem
  Vj : Scope
  Z : Scope
  Pj : Outport
  qj : Outport  Port=2
  wires:
  Rate-Deoxy-Hemo/1(qj) -> qj/1
  Zj/1 -> Vasodilatory Signal/1(Zj), Z/1
  Vasodilatory Signal/1(Sj) -> Sj/1
  Rate Blood Volume/2(Fjout) -> Fjout/1, Rate-Total-Hemo/2(Fjout), Rate-Deoxy-Hemo/3(Fjout)  "Fjout"
  Rate Blood Volume/1(Vj) -> Vj/1, Rate-Total-Hemo/1(Vj), Rate-Deoxy-Hemo/2(Vj)  "Vj"
  Rate-Total-Hemo/1(Pj) -> Pj/1
  Efp/1(Efp) -> Rate-Deoxy-Hemo/4(Efp), Efp_1/1  "Efp"
  Vasodilatory Signal/2(Fjin) -> Efp/1(fjin), Fjin_1/1, Rate-Total-Hemo/3(Fjin), Rate-Deoxy-Hemo/1(Fjin), Rate Blood Volume/1(Fjin)  "Fjin"

== system Neurofeedback_Fuzzy_MISO_Full_3x3/Synthetic Human Agent1/Human_Pressure ==
  Zt : Inport
  Clock : Clock
  Gain : Gain  Gain=10
  Pressure Generator : MATLAB Function  TreatAsAtomicUnit=on
  SENSOR : MATLAB Function  TreatAsAtomicUnit=on
  Scope : Scope
  Scope1 : Scope
  Pobs : Outport
  wires:
  Clock/1 -> Pressure Generator/2(t)
  Zt/1 -> Pressure Generator/1(Zt)
  SENSOR/1(Pobs) -> Scope1/1, Gain/1
  Pressure Generator/1(Pobs) -> SENSOR/1(Vout), Scope/1
  Gain/1 -> Pobs/1

== system Neurofeedback_Fuzzy_MISO_Full_3x3/Synthetic Human Agent1/Neurodynamics_Static ==
  U : Inport
  C : Inport  Port=2
  B : Inport  Port=3
  A : Inport  Port=4
  B_Dynamic1 : Subsystem
  Clock : Clock
  Integrator : Integrator
  Jt : MATLAB Function  TreatAsAtomicUnit=on
  Product1 : Product  Multiplication=Matrix(*)
  Sum : Sum  Inputs=|++
  Z : Outport
  New B : Outport  Port=2
  wires:
  Integrator/1 -> Z/1, Jt/1(Zt)
  B_Dynamic1/1(B_d) -> New B/1, Jt/3(B_input)
  A/1 -> Jt/4(A_input)
  U/1 -> Product1/2, B_Dynamic1/1(U), Jt/2(U)
  Sum/1 -> Integrator/1
  Clock/1 -> B_Dynamic1/3(T)
  B/1 -> B_Dynamic1/2(B)
  Jt/1(Jt) -> Sum/2
  Product1/1 -> Sum/1
  C/1 -> Product1/1

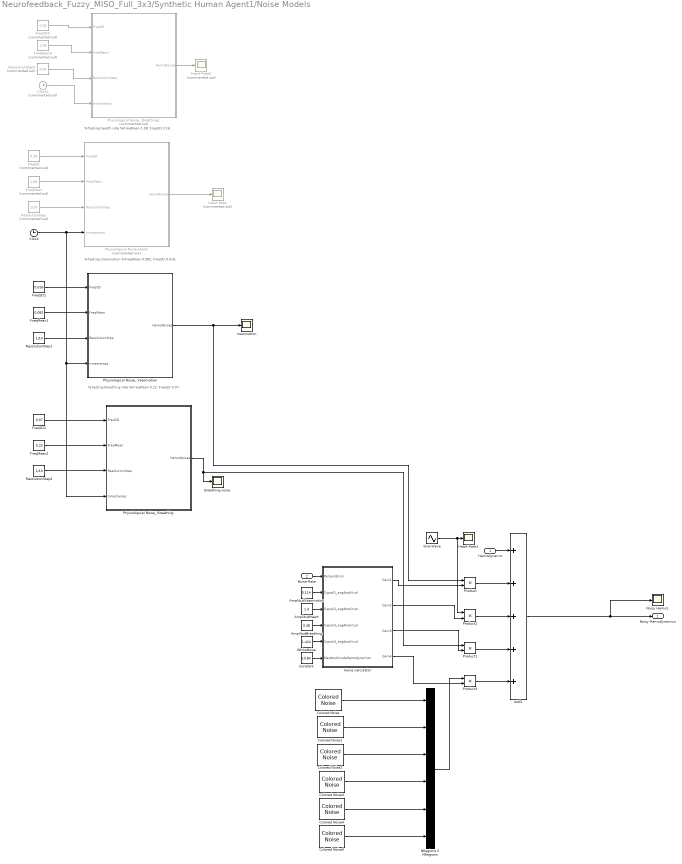
== system Neurofeedback_Fuzzy_MISO_Full_3x3/Synthetic Human Agent1/Noise Models ==
  note: %Testing hearth rate
      | %FreqMean 1.08; FreqSD 0.16;
  note: %Testing Breathing rate
      | %FreqMean 0.22; FreqSD 0.07;
  note: %Testing Vasomotion
      | %FreqMean 0.082; FreqSD 0.016;
  Hemodynamic : Inport
  Noise-Rate : Inport  Port=2
  Add1 : Sum  Inputs=+++++
  AmplitudBreathing : Constant  Value=0.36
  AmplitudHeart : Constant  Value=1.4
  AmplitudVasomotion : Constant  Value=0.114
  Breathing noise : Scope
  Clock : Clock
  Clock1 : Clock  Commented=on
  Colored Noise : dspsrcs4/Colored Noise  Color=white  InverseFrequencyPower=1  BoundedOutput=on  NumChannels=1  OutputDataType=double  SamplesPerFrame=1  SampleTime=1/10  RandomStream=mt19937ar with seed  Seed=67  SimulateUsing=Interpreted execution
      settings: SourceProductBaseCode=DS
  Colored Noise1 : dspsrcs4/Colored Noise  Color=white  InverseFrequencyPower=1  BoundedOutput=on  NumChannels=1  OutputDataType=double  SamplesPerFrame=1  SampleTime=1/10  RandomStream=mt19937ar with seed  Seed=40  SimulateUsing=Interpreted execution
      settings: SourceProductBaseCode=DS
  Colored Noise2 : dspsrcs4/Colored Noise  Color=white  InverseFrequencyPower=1  BoundedOutput=on  NumChannels=1  OutputDataType=double  SamplesPerFrame=1  SampleTime=1/10  RandomStream=mt19937ar with seed  Seed=41  SimulateUsing=Interpreted execution
      settings: SourceProductBaseCode=DS
  Colored Noise3 : dspsrcs4/Colored Noise  Color=white  InverseFrequencyPower=1  BoundedOutput=on  NumChannels=1  OutputDataType=double  SamplesPerFrame=1  SampleTime=1/10  RandomStream=mt19937ar with seed  Seed=50  SimulateUsing=Interpreted execution
      settings: SourceProductBaseCode=DS
  Colored Noise4 : dspsrcs4/Colored Noise  Color=white  InverseFrequencyPower=1  BoundedOutput=on  NumChannels=1  OutputDataType=double  SamplesPerFrame=1  SampleTime=1/10  RandomStream=mt19937ar with seed  Seed=50  SimulateUsing=Interpreted execution
      settings: SourceProductBaseCode=DS
  Colored Noise5 : dspsrcs4/Colored Noise  Color=white  InverseFrequencyPower=1  BoundedOutput=on  NumChannels=1  OutputDataType=double  SamplesPerFrame=1  SampleTime=1/10  RandomStream=mt19937ar with seed  Seed=50  SimulateUsing=Interpreted execution
      settings: SourceProductBaseCode=DS
  Constant : Constant  Value=10.84
  FreqMean : Constant  Commented=on  Value=1.08
  FreqMean1 : Constant  Value=0.082
  FreqMean2 : Constant  Value=0.22
  FreqMean3 : Constant  Commented=on  Value=1.08
  FreqSD : Constant  Commented=on  Value=0.16
  FreqSD1 : Constant  Value=0.016
  FreqSD2 : Constant  Value=0.07
  FreqSD3 : Constant  Commented=on  Value=0.16
  Gains calculator : MATLAB Function  TreatAsAtomicUnit=on
  Heart Rate : Scope  Commented=on
  Heart Rate1 : Scope
  Heart Rate2 : Scope  Commented=on
  NRegions X NRegions : Mux  Inputs=6
  Noisy Hemo1 : Scope
  Physiological Noise_ Breathing : MATLAB Function  TreatAsAtomicUnit=on
  Physiological Noise_ Breathing1 : MATLAB Function  Commented=on  TreatAsAtomicUnit=on
  Physiological Noise_ Vasomotion : MATLAB Function  TreatAsAtomicUnit=on
  Physiological Noise_Heart : MATLAB Function  Commented=on  TreatAsAtomicUnit=on
  Product{,1..3} (4 alike) : Product
  ResolutionStep : Constant  Commented=on  Value=1/10
  ResolutionStep1 : Constant  Value=1/10
  ResolutionStep2 : Constant  Value=1/10
  ResolutionStep3 : Constant  Commented=on  Value=1/10
  Sine Wave : Sin  Frequency=1.08 * 2*pi  SampleTime=0
  Vasomotion : Scope
  WhiteNoise : Constant  Value=1.424
  Noisy Hemodynamics : Outport
  wires:
  FreqSD/1 -> Physiological Noise_Heart/1(FreqSD)
  FreqMean/1 -> Physiological Noise_Heart/2(FreqMean)
  ResolutionStep/1 -> Physiological Noise_Heart/3(ResolutionStep)
  ResolutionStep1/1 -> Physiological Noise_ Vasomotion/3(ResolutionStep)
  FreqSD1/1 -> Physiological Noise_ Vasomotion/1(FreqSD)
  Clock/1 -> Physiological Noise_Heart/4(timestamps), Physiological Noise_ Breathing/4(timestamps), Physiological Noise_ Vasomotion/4(timestamps)
  FreqMean1/1 -> Physiological Noise_ Vasomotion/2(FreqMean)
  Physiological Noise_ Breathing/1(HemoNoises) -> Product1/1, Breathing noise/1
  ResolutionStep2/1 -> Physiological Noise_ Breathing/3(ResolutionStep)
  FreqMean2/1 -> Physiological Noise_ Breathing/2(FreqMean)
  FreqSD2/1 -> Physiological Noise_ Breathing/1(FreqSD)
  Physiological Noise_ Vasomotion/1(HemoNoises) -> Product/1, Vasomotion/1
  Physiological Noise_Heart/1(HemoNoises) -> Heart Rate/1
  Physiological Noise_ Breathing1/1(HemoNoises) -> Heart Rate2/1
  Clock1/1 -> Physiological Noise_ Breathing1/4(timestamps)
  FreqSD3/1 -> Physiological Noise_ Breathing1/1(FreqSD)
  FreqMean3/1 -> Physiological Noise_ Breathing1/2(FreqMean)
  ResolutionStep3/1 -> Physiological Noise_ Breathing1/3(ResolutionStep)
  Sine Wave/1 -> Product2/1, Heart Rate1/1
  Gains calculator/1(Gain1) -> Product/2
  Noise-Rate/1 -> Gains calculator/1(PercentError)
  Add1/1 -> Noisy Hemodynamics/1, Noisy Hemo1/1
  AmplitudVasomotion/1 -> Gains calculator/2(Signal1_avgAmplitud)
  Hemodynamic/1 -> Add1/1
  Constant/1 -> Gains calculator/6(MaxAmplitudeHemodynamics)
  Gains calculator/2(Gain2) -> Product2/2
  Gains calculator/3(Gain3) -> Product1/2
  AmplitudHeart/1 -> Gains calculator/3(Signal2_avgAmplitud)
  AmplitudBreathing/1 -> Gains calculator/4(Signal3_avgAmplitud)
  Colored Noise/1 -> NRegions X NRegions/1
  Colored Noise1/1 -> NRegions X NRegions/2
  Colored Noise2/1 -> NRegions X NRegions/3
  Colored Noise3/1 -> NRegions X NRegions/4
  WhiteNoise/1 -> Gains calculator/5(Signal4_avgAmplitud)
  Gains calculator/4(Gain4) -> Product3/2
  NRegions X NRegions/1 -> Product3/1
  Product/1 -> Add1/2
  Product2/1 -> Add1/3
  Product1/1 -> Add1/4
  Product3/1 -> Add1/5
  Colored Noise4/1 -> NRegions X NRegions/5
  Colored Noise5/1 -> NRegions X NRegions/6

== system Neurofeedback_Fuzzy_MISO_Full_3x3/fNIRS Processing/RC High pass ==
  Hemodynamics : Inport
  Add : Sum  Inputs=+-
  Discrete Derivative : simulink/Discrete/Discrete Derivative  gainval=0.1  ICPrevScaledInput=0.0  OutMin=[]  OutMax=[]  OutDataType=fixdt(1, 16)  OutScaling=2^-10  DoSatur=off
  Discrete Derivative1 : simulink/Discrete/Discrete Derivative  gainval=0.12  ICPrevScaledInput=0.0  OutMin=[]  OutMax=[]  OutDataType=fixdt(1, 16)  OutScaling=2^-10  DoSatur=off
  Gain : Gain  Gain=800
  u : Outport
  wires:
  Add/1 -> Gain/1
  Gain/1 -> Discrete Derivative/1, u/1
  Discrete Derivative/1 -> Add/2
  Discrete Derivative1/1 -> Add/1
  Hemodynamics/1 -> Discrete Derivative1/1

== system Neurofeedback_Fuzzy_MISO_Full_3x3/fNIRS Processing/RC High pass1 ==
  Hemodynamics : Inport
  Add : Sum  Inputs=+-
  Discrete Derivative : simulink/Discrete/Discrete Derivative  gainval=1.2  ICPrevScaledInput=0.0  OutMin=[]  OutMax=[]  OutDataType=fixdt(1, 16)  OutScaling=2^-10  DoSatur=off
  Discrete Derivative1 : simulink/Discrete/Discrete Derivative  gainval=1.4  ICPrevScaledInput=0.0  OutMin=[]  OutMax=[]  OutDataType=fixdt(1, 16)  OutScaling=2^-10  DoSatur=off
  Gain : Gain  Gain=800
  Out1 : Outport
  wires:
  Add/1 -> Gain/1
  Gain/1 -> Discrete Derivative/1, Out1/1
  Discrete Derivative/1 -> Add/2
  Discrete Derivative1/1 -> Add/1
  Hemodynamics/1 -> Discrete Derivative1/1

== system Neurofeedback_Fuzzy_MISO_Full_3x3/fNIRS Processing/RC Low pass ==
  Hemodynamics : Inport
  Add : Sum  Inputs=+-
  Discrete Derivative : simulink/Discrete/Discrete Derivative  gainval=3.2  ICPrevScaledInput=0.0  OutMin=[]  OutMax=[]  OutDataType=fixdt(1, 16)  OutScaling=2^-10  DoSatur=off
  Out1 : Outport
  wires:
  Hemodynamics/1 -> Add/1
  Discrete Derivative/1 -> Add/2
  Add/1 -> Discrete Derivative/1, Out1/1

== system Neurofeedback_Fuzzy_MISO_Full_3x3/Subsystem/Incremental_Avg_Boot1/Reboot ==
  Cycle_time : Inport
  periods : Inport  Port=2
  Clock1 : Clock
  Constant1 : Constant
  Delay1 : Delay  DelayLength=1
  Divide : Product  Inputs=*/
  MATLAB Function1 : MATLAB Function  TreatAsAtomicUnit=on
  MATLAB Function2 : MATLAB Function  TreatAsAtomicUnit=on
  Timer : Display
  Timer1 : Display
  y : Outport
  Time : Outport  Port=2
  wires:
  MATLAB Function1/1(Reset) -> MATLAB Function2/1(reset), Timer1/1
  MATLAB Function2/1(y) -> y/1, Divide/1, Delay1/1
  Constant1/1 -> Divide/2
  Clock1/1 -> MATLAB Function1/1(Timer), Timer/1
  periods/1 -> MATLAB Function1/3(periods)
  Delay1/1 -> MATLAB Function2/2(y_s)
  Divide/1 -> Time/1
  Cycle_time/1 -> MATLAB Function1/2(Cycle_time)

== system Neurofeedback_Fuzzy_MISO_Full_3x3/Synthetic Human Agent/Hemodynamics/Rate Blood Volume ==
  Fjin : Inport
  Add : Sum  Inputs=+-
  Add1 : Sum
  Divide : Product  Inputs=*/
  Fv_s : MATLAB Function  TreatAsAtomicUnit=on
  Integrator : Integrator  InitialCondition=exp([0;0])
  Product : Product
  Scope : Scope
  Tjv : Constant  Value=2*exp([0;1])
  Vj/Tjv : MATLAB Function  TreatAsAtomicUnit=on
  Vj : Outport
  Fjout : Outport  Port=2
  wires:
  Fjin/1 -> Add/1
  Integrator/1 -> Vj/1, Vj/Tjv/1(Vj), Fv_s/1(Vj)  "Vj"
  Divide/1 -> Product/2, Integrator/1
  Fv_s/1(Vj_expphi) -> Add/2, Add1/1
  Add/1 -> Divide/1
  Vj/Tjv/1(Vj_Tjv) -> Divide/2
  Product/1 -> Add1/2
  Tjv/1 -> Product/1
  Add1/1 -> Scope/1, Fjout/1

== system Neurofeedback_Fuzzy_MISO_Full_3x3/Synthetic Human Agent/Hemodynamics/Rate-Deoxy-Hemo ==
  Fjin : Inport
  Vj : Inport  Port=2
  Fjout : Inport  Port=3
  Efp : Inport  Port=4
  Divide : Product  Inputs=*/
  Integrator : Integrator  InitialCondition=exp([0;0])
  Product : Product
  Product1 : Product
  Subtract : Sum  Inputs=+-
  qj_scope : Scope
  qj : Outport
  wires:
  Efp/1 -> Product/2
  Divide/1 -> Product1/2
  Subtract/1 -> Integrator/1
  Integrator/1 -> qj/1, Divide/1, qj_scope/1
  Vj/1 -> Divide/2
  Product1/1 -> Subtract/2
  Fjin/1 -> Product/1
  Fjout/1 -> Product1/1
  Product/1 -> Subtract/1

== system Neurofeedback_Fuzzy_MISO_Full_3x3/Synthetic Human Agent/Hemodynamics/Rate-Total-Hemo ==
  Vj : Inport
  Fjout : Inport  Port=2
  Fjin : Inport  Port=3
  Divide : Product  Inputs=*/
  Integrator : Integrator  InitialCondition=exp([0;0])
  Product : Product
  Subtract : Sum  Inputs=+-
  pj : Scope
  Pj : Outport
  wires:
  Fjout/1 -> Subtract/2
  Product/1 -> Integrator/1
  Vj/1 -> Divide/2
  Subtract/1 -> Product/1
  Fjin/1 -> Subtract/1
  Divide/1 -> Product/2
  Integrator/1 -> Pj/1, pj/1, Divide/1

== system Neurofeedback_Fuzzy_MISO_Full_3x3/Synthetic Human Agent/Hemodynamics/Vasodilatory Signal ==
  Zj : Inport
  Add : Sum  Inputs=+--
  Add1 : Sum  Inputs=+-
  Constant1 : Constant
  Integrator : Integrator
  Integrator1 : Integrator  InitialCondition=exp([0;0])
  K : Gain  Gain=0.64*exp([0;0.05])
  Scope1 : Scope
  Yj : Gain  Gain=0.32*exp([0;0.05])
  Sj : Outport
  Fjin : Outport  Port=2
  wires:
  Add1/1 -> Yj/1
  K/1 -> Add/2  "Kj*Sj"
  Constant1/1 -> Add1/2
  Zj/1 -> Add/1
  Integrator1/1 -> Fjin/1, Scope1/1, Add1/1
  Integrator/1 -> Sj/1, K/1, Integrator1/1
  Add/1 -> Integrator/1
  Yj/1 -> Add/3  "Yj(Fjin - 1)"

== system Neurofeedback_Fuzzy_MISO_Full_3x3/Synthetic Human Agent/Neurodynamics_Static/B_Dynamic ==
  U : Inport
  B : Inport  Port=2
  T : Inport  Port=3
  Delay : Delay  DelayLength=1  InitialCondition=0
  Display : Display
  Display1 : Display
  Display2 : Display
  MATLAB Function : MATLAB Function  TreatAsAtomicUnit=on
  B_d : Outport
  wires:
  MATLAB Function/2(Th) -> Delay/1, Display1/1
  B/1 -> MATLAB Function/1(B)
  MATLAB Function/1(B_d) -> Display/1, B_d/1
  Delay/1 -> MATLAB Function/4(Th_O)
  T/1 -> MATLAB Function/3(T)
  U/1 -> MATLAB Function/2(U), Display2/1

== system Neurofeedback_Fuzzy_MISO_Full_3x3/Synthetic Human Agent1/Hemodynamics/Rate Blood Volume ==
  Fjin : Inport
  Add : Sum  Inputs=+-
  Add1 : Sum
  Divide : Product  Inputs=*/
  Fv_s : MATLAB Function  TreatAsAtomicUnit=on
  Integrator : Integrator  InitialCondition=exp([0;0;0])
  Product : Product
  Scope : Scope
  Tjv : Constant  Value=2*exp([0;1;0])
  Vj/Tjv : MATLAB Function  TreatAsAtomicUnit=on
  Vj : Outport
  Fjout : Outport  Port=2
  wires:
  Fjin/1 -> Add/1
  Integrator/1 -> Vj/1, Vj/Tjv/1(Vj), Fv_s/1(Vj)  "Vj"
  Divide/1 -> Product/2, Integrator/1
  Fv_s/1(Vj_expphi) -> Add/2, Add1/1
  Add/1 -> Divide/1
  Vj/Tjv/1(Vj_Tjv) -> Divide/2
  Product/1 -> Add1/2
  Tjv/1 -> Product/1
  Add1/1 -> Scope/1, Fjout/1

== system Neurofeedback_Fuzzy_MISO_Full_3x3/Synthetic Human Agent1/Hemodynamics/Rate-Deoxy-Hemo ==
  Fjin : Inport
  Vj : Inport  Port=2
  Fjout : Inport  Port=3
  Efp : Inport  Port=4
  Divide : Product  Inputs=*/
  Integrator : Integrator  InitialCondition=exp([0;0;0])
  Product : Product
  Product1 : Product
  Subtract : Sum  Inputs=+-
  qj_scope : Scope
  qj : Outport
  wires:
  Efp/1 -> Product/2
  Divide/1 -> Product1/2
  Subtract/1 -> Integrator/1
  Integrator/1 -> qj/1, Divide/1, qj_scope/1
  Vj/1 -> Divide/2
  Product1/1 -> Subtract/2
  Fjin/1 -> Product/1
  Fjout/1 -> Product1/1
  Product/1 -> Subtract/1

== system Neurofeedback_Fuzzy_MISO_Full_3x3/Synthetic Human Agent1/Hemodynamics/Rate-Total-Hemo ==
  Vj : Inport
  Fjout : Inport  Port=2
  Fjin : Inport  Port=3
  Divide : Product  Inputs=*/
  Integrator : Integrator  InitialCondition=exp([0;0;0])
  Product : Product
  Subtract : Sum  Inputs=+-
  pj : Scope
  Pj : Outport
  wires:
  Fjout/1 -> Subtract/2
  Product/1 -> Integrator/1
  Vj/1 -> Divide/2
  Subtract/1 -> Product/1
  Fjin/1 -> Subtract/1
  Divide/1 -> Product/2
  Integrator/1 -> Pj/1, pj/1, Divide/1

== system Neurofeedback_Fuzzy_MISO_Full_3x3/Synthetic Human Agent1/Hemodynamics/Vasodilatory Signal ==
  Zj : Inport
  Add : Sum  Inputs=+--
  Add1 : Sum  Inputs=+-
  Constant1 : Constant
  Integrator : Integrator
  Integrator1 : Integrator  InitialCondition=exp([0;0;0])
  K : Gain  Gain=0.64*exp([0;0.05;0.05])
  Scope1 : Scope
  Yj : Gain  Gain=0.32*exp([0;0.05;0.05])
  Sj : Outport
  Fjin : Outport  Port=2
  wires:
  Add1/1 -> Yj/1
  K/1 -> Add/2  "Kj*Sj"
  Constant1/1 -> Add1/2
  Zj/1 -> Add/1
  Integrator1/1 -> Fjin/1, Scope1/1, Add1/1
  Integrator/1 -> Sj/1, K/1, Integrator1/1
  Add/1 -> Integrator/1
  Yj/1 -> Add/3  "Yj(Fjin - 1)"

== system Neurofeedback_Fuzzy_MISO_Full_3x3/Synthetic Human Agent1/Neurodynamics_Static/B_Dynamic1 ==
  U : Inport
  B : Inport  Port=2
  T : Inport  Port=3
  Delay : Delay  DelayLength=1  InitialCondition=0
  Display : Display
  Display1 : Display
  Display2 : Display
  MATLAB Function : MATLAB Function  TreatAsAtomicUnit=on
  B_d : Outport
  wires:
  MATLAB Function/2(Th) -> Delay/1, Display1/1
  B/1 -> MATLAB Function/1(B)
  MATLAB Function/1(B_d) -> Display/1, B_d/1
  Delay/1 -> MATLAB Function/4(Th_O)
  T/1 -> MATLAB Function/3(T)
  U/1 -> MATLAB Function/2(U), Display2/1

== matlab function Neurofeedback_Fuzzy_MISO_Full_3x3/Synthetic Human Agent/Noise Models/Gains calculator ==
  settings: updateMethod=DISCRETE
  data: PercentError input; Signal1_avgAmplitud input; Signal2_avgAmplitud input; Signal3_avgAmplitud input; Signal4_avgAmplitud input; Gain1 output; MaxAmplitudeHemodynamics input; Gain2 output; Gain3 output; Gain4 output
function [Gain1, Gain2, Gain3, Gain4]    = Noise_gains(PercentError, Signal1_avgAmplitud,Signal2_avgAmplitud ,Signal3_avgAmplitud,Signal4_avgAmplitud,MaxAmplitudeHemodynamics)

Gain1 = ((MaxAmplitudeHemodynamics / 100) * PercentError)/ Signal1_avgAmplitud;

Gain2 = ((MaxAmplitudeHemodynamics / 100) * PercentError)/ Signal2_avgAmplitud;

Gain3 = ((MaxAmplitudeHemodynamics / 100) * PercentError)/ Signal3_avgAmplitud;

Gain4 = ((MaxAmplitudeHemodynamics / 100) * PercentError)/ Signal4_avgAmplitud;

== matlab function Neurofeedback_Fuzzy_MISO_Full_3x3/fNIRS Processing/Channel Organizer1 ==
  data: u input; y1 output; y2 output; y3 output
function [y1,y2, y3]= fcn(u)

y1 = [1; 2;];
y2 = [3; 4;];
y3 = [4; 6;];

y1(1) = u(1,1);
y1(2) = u(1,2);

y2(1) = u(2,1);
y2(2) = u(2,2);

y3(1) = u(3,1);
y3(2) = u(3,2);

== matlab function Neurofeedback_Fuzzy_MISO_Full_3x3/Synthetic Human Agent/Noise Models/Physiological Noise_ Breathing ==
  settings: updateMethod=DISCRETE
  data: FreqSD input; HemoNoises output; FreqMean input; ResolutionStep input; timestamps input
function HemoNoises  = Neurofeedback_PhysiologicalNoise(FreqSD, FreqMean, ResolutionStep, timestamps)
%% Version V1
% Authors - Mario De Los Santos, Felipe Orihuela-Espina, Javier
% Herrera-Vega, Javier Andreu-Pérez
% Date - July 18th, 2022
% Email - madlsh3517@gmail.com
% Based on: Elwell et. al., 1999. Oscillations in cerebal haemodynamics.
%
%% Input Parameters
% FreqSD - Frequency standard deviation of the physiological noise. Scalar
% FreqMean - Frequency Mean of the physiological noise. Scalar
% Resolution Step - Sampling rate. Scalar
% Timestamps - Time sequence for the stimulus train. <1 x simulationLength>
% NRegions - Number of regions activated. Scalar.
%% Output Parameters
% 
% HemoNoises -  Noise generation for the hemodynamics signals.
%               <NRegions x simulationLength>
%
%% 

%Variables to ADD the noises to the models. 
% These variables divide the hemodynamics 
% inputs depending on the number of regions.
HemoNoises = 0;

%Calculation of the operative ranges to use
Initial =  FreqMean - 2 * FreqSD;
Ending = FreqMean + 2 * FreqSD;
Calsize =  (Ending - Initial - ResolutionStep)/ResolutionStep;
FrequencySet = linspace(Initial, Ending, Calsize);

amplitudeScaling = 1;
for i = 1:Calsize
    s = rng; %Rebot random seeed 
    %Random Amplitude
    %Centralized gaussian in the dispersion mean 
    %A = 0;
    L = normrnd(FreqMean, FreqSD);
    A = amplitudeScaling * L;
  
    %Random phase
    theta = (2 * pi * L - pi );
  
    %Fundamental signal
    tmpSin = A * sin(pi * FrequencySet(1,i) * timestamps + theta);
    HemoNoises = HemoNoises + tmpSin;
end
%This section should be generalized but do the work for now.

== matlab function Neurofeedback_Fuzzy_MISO_Full_3x3/Synthetic Human Agent/Visual Interpretation ==
  data: Visual_Stimulus input; Response output; t input
function Response = fcn(Visual_Stimulus, t)
    R=17.5; %Resistor [Ohms] 10k 
    C= 0.65; %Capacitor [Faradays] 1mF
    V= Visual_Stimulus; %Voltage or system reference;
    Vc = V * (1- exp(-t/(R*C))); % Voltage at the capacitor  
    
Response = Vc;

== matlab function Neurofeedback_Fuzzy_MISO_Full_3x3/Synthetic Human Agent1/DH and DQ/MATLAB Function1 ==
  data: DH1 input; H output; DH2 input; DQ1 input; DQ2 input
function H = hemo(DH1, DH2, DQ1, DQ2)
H = zeros(1,4);

H(1,1) = DQ1;
H(1,2) = DQ2;
H(1,3) = DH1;
H(1,4) = DH2;

== matlab function Neurofeedback_Fuzzy_MISO_Full_3x3/Synthetic Human Agent1/Hemodynamics/Efp ==
  data: fjin input; Efp output
function Efp= fcn(fjin)

Efp = (1 - (1 - 0.32).^ (1 ./ fjin))/0.32;

== matlab function Neurofeedback_Fuzzy_MISO_Full_3x3/Synthetic Human Agent/Noise Models/Physiological Noise_ Breathing1 ==
  settings: updateMethod=DISCRETE
  data: FreqSD input; HemoNoises output; FreqMean input; ResolutionStep input; timestamps input
function HemoNoises  = Neurofeedback_PhysiologicalNoise(FreqSD, FreqMean, ResolutionStep, timestamps)
%% Version V1
% Authors - Mario De Los Santos, Felipe Orihuela-Espina, Javier
% Herrera-Vega, Javier Andreu-Pérez
% Date - July 18th, 2022
% Email - madlsh3517@gmail.com
% Based on: Elwell et. al., 1999. Oscillations in cerebal haemodynamics.
%
%% Input Parameters
% FreqSD - Frequency standard deviation of the physiological noise. Scalar
% FreqMean - Frequency Mean of the physiological noise. Scalar
% Resolution Step - Sampling rate. Scalar
% Timestamps - Time sequence for the stimulus train. <1 x simulationLength>
% NRegions - Number of regions activated. Scalar.
%% Output Parameters
% 
% HemoNoises -  Noise generation for the hemodynamics signals.
%               <NRegions x simulationLength>
%
%% 

%Variables to ADD the noises to the models. 
% These variables divide the hemodynamics 
% inputs depending on the number of regions.
HemoNoises = 0;

%Calculation of the operative ranges to use
Initial =  FreqMean - 2 * FreqSD;
Ending = FreqMean + 2 * FreqSD;
Calsize =  (Ending - Initial)/ResolutionStep;
FrequencySet = linspace(Initial, Ending, Calsize);

amplitudeScaling = 1;
for i = 1:Calsize
    s = rng; %Rebot random seeed 
    %Random Amplitude
    %Centralized gaussian in the dispersion mean 
    %A = 0;
    L = normrnd(FreqMean, FreqSD);
    A = amplitudeScaling * L;
  
    %Random phase
    theta = 0;
  
    %Fundamental signal
    tmpSin = A * sin((pi * FrequencySet(1,i) * timestamps + theta)*2*pi);
    HemoNoises = HemoNoises + tmpSin;
end
%This section should be generalized but do the work for now.
